simulink model "VSI_SPWM_FOC"  (R2020b)
settings: Solver=FixedStepDiscrete  StartTime=0.0  StopTime=0.02  RelTol=1e-3
libraries: powerlib x16, pid_lib x3, simulink x3, powerlib_meascontrol x1
settings Model: Creator=90554  LastModifiedBy=90554

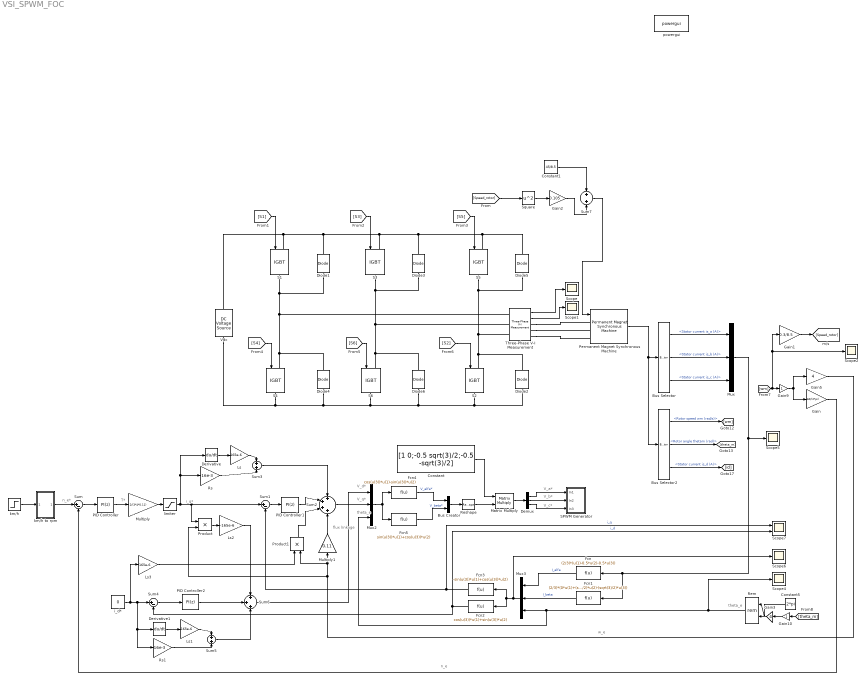
== system VSI_SPWM_FOC ==
  note: V_c*
  note: V_b*
  note: V_a*
  note: theta_e
  note: flux linkage
  note: n_e*
  note: T*
  note: i_q*
  note: V_q*
  note: V_d*
  note: n_e
  note: w_e
  note: theta_e
  Bus Creator : BusCreator  Inputs=2
  Bus Selector : BusSelector  OutputSignals=Stator current is_a (A),Stator current is_b (A),Stator current is_c (A)
  Bus Selector2 : BusSelector  OutputSignals=Rotor speed wm (rad/s),Rotor angle thetam (rad),Stator current is_d (A)
  Constant : Constant  Value=[1 0;-0.5 sqrt(3)/2;-0.5 -sqrt(3)/2]  VectorParams1D=off
  Constant1 : Constant  Value=45/8.5
  Constant5 : Constant  Value=2*pi
  Demux : Demux  Outputs=3
  Derivative : Derivative
  Derivative1 : Derivative
  Diode{1..6} (6 alike) : powerlib/Power Electronics/Diode  Ron=0.001  Lon=0  Vf=0.8  IC=0  UseSnubber=0  Rs=inf  Cs=0  Measurements=off
  Fcn : Fcn  Expr=(2/3)*(u(1)-0.5*u(2)-0.5*u(3))
  Fcn1 : Fcn  Expr=(2/3)*(0*u(1)+(sqrt(3)/2)*u(2)-(sqrt(3)/2)*u(3))
  Fcn2 : Fcn  Expr=cos(u(3))*u(1)+sin(u(3))*u(2)
  Fcn3 : Fcn  Expr=-sin(u(3))*u(1)+cos(u(3))*u(2)
  Fcn4 : Fcn  Expr=cos(u(3))*u(1)-sin(u(3))*u(2)
  Fcn5 : Fcn  Expr=sin(u(3))*u(1)+cos(u(3))*u(2)
  Gain : Gain  Gain=60/(2*pi)
  Gain1 : Gain  Gain=0.3/8.5
  Gain10 : Gain
  Gain2 : Gain  Gain=0.105
  Gain3 : Gain  Gain=4
  Gain5 : Gain  Gain=4
  Gain9 : Gain
  Ls : Gain  Gain=165e-6
  Ls1 : Gain  Gain=165e-6
  Ls2 : Gain  Gain=-165e-6
  Ls3 : Gain  Gain=165e-6
  Matrix Multiply : Product  Multiplication=Matrix(*)
  Multiply : Gain  Gain=2/(3*4*0.11)
  Multiply1 : Gain  Gain=0.11
  Mux : Mux  Inputs=3
  Mux2 : Mux  Inputs=3
  Mux3 : Mux  Inputs=3
  PID Controller : pid_lib/PID Controller  Controller=PI  Form=Parallel  TimeDomain=Discrete-time  UseExternalTs=off  SampleTime=-1  IntegratorMethod=Forward Euler  FilterMethod=Forward Euler  ControllerParametersSource=internal  P=5  I=1  D=0  UseFilter=on  N=100  TunerSelectOption=Transfer Function Based (PID Tuner App)  InitialConditionSource=internal  InitialConditionForIntegrator=0  InitialConditionForFilter=0  DifferentiatorICPrevScaledInput=0  ExternalReset=none  TrackingMode=off  Kt=1  LimitOutput=off  SatLimitsSource=internal  UpperSaturationLimit=inf  LowerSaturationLimit=-inf  LinearizeAsGain=on  AntiWindupMode=none  Kb=1  POutMin=[]  POutMax=[]  IOutMin=[]  IOutMax=[]  DOutMin=[]  DOutMax=[]  NOutMin=[]  NOutMax=[]  SumOutMin=[]  SumOutMax=[]  SaturationOutMin=[]  SaturationOutMax=[]  PParamMin=[]  PParamMax=[]  IParamMin=[]  IParamMax=[]  DParamMin=[]  DParamMax=[]  NParamMin=[]  NParamMax=[]  KbParamMin=[]  KbParamMax=[]  KtParamMin=[]  KtParamMax=[]  KbOutMin=[]  KbOutMax=[]  KtOutMin=[]  KtOutMax=[]  IntegratorOutMin=[]  IntegratorOutMax=[]  FilterOutMin=[]  FilterOutMax=[]  SumI1OutMin=[]  SumI1OutMax=[]  SumI2OutMin=[]  SumI2OutMax=[]  SumI3OutMin=[]  SumI3OutMax=[]  SumI4OutMin=[]  SumI4OutMax=[]  SumDOutMin=[]  SumDOutMax=[]  DifferentiatorOutMin=[]  DifferentiatorOutMax=[]  FilterDiffOutCoefMin=[]  FilterDiffOutCoefMax=[]  ReciprocalOutMin=[]  ReciprocalOutMax=[]  SumDenOutMin=[]  SumDenOutMax=[]  SumNumOutMin=[]  SumNumOutMax=[]  DivideOutMin=[]  DivideOutMax=[]  UdiffTsProdOutMin=[]  UdiffTsProdOutMax=[]  NTsProdOutMin=[]  NTsProdOutMax=[]  UintegralTsProdOutMin=[]  UintegralTsProdOutMax=[]  UngainTsProdOutMin=[]  UngainTsProdOutMax=[]  IntegratorContinuousStateAttributes=''  IntegratorStateMustResolveToSignalObject=off  IntegratorRTWStateStorageClass=Auto  FilterContinuousStateAttributes=''  FilterStateMustResolveToSignalObject=off  FilterRTWStateStorageClass=Auto  ParallelPVariant=InternalParameters  IdealPVariant=Disabled  IVariant=InternalParameters  DVariant=Disabled  IntegratorVariant=Discrete  SatVariant=Disabled  AWVariant=Passthrough  PCopyVariant=Disabled  TRVariant=Disabled  FdbkBlocksVariant=Forward  IdealPFdbkVariant=Disabled  SatFdbkVariant=Disabled  DerivativeFilterVariant=Disabled  NVariant=Disabled  NCopyVariant=Disabled_SignalSpec  FilterICVariant=Disabled  IntegratorICVariant=InternalICs  ExternalResetVariant=Disabled  TRSumVariant=Passthrough  SumFdbkVariant=Disabled  SumVariant=Sum_PI  TsampFilterVariant=InternalTs  TsampNgainVariant=Passthrough  TsampIntegralVariant=Passthrough  ExternalSaturationOutDataTypeStr=Inherit: Same as second input
  PID Controller1 : pid_lib/PID Controller  Controller=PI  Form=Parallel  TimeDomain=Discrete-time  UseExternalTs=off  SampleTime=-1  IntegratorMethod=Forward Euler  FilterMethod=Forward Euler  ControllerParametersSource=internal  P=5  I=1  D=0  UseFilter=on  N=100  TunerSelectOption=Transfer Function Based (PID Tuner App)  InitialConditionSource=internal  InitialConditionForIntegrator=0  InitialConditionForFilter=0  DifferentiatorICPrevScaledInput=0  ExternalReset=none  TrackingMode=off  Kt=1  LimitOutput=off  SatLimitsSource=internal  UpperSaturationLimit=inf  LowerSaturationLimit=-inf  LinearizeAsGain=on  AntiWindupMode=none  Kb=1  POutMin=[]  POutMax=[]  IOutMin=[]  IOutMax=[]  DOutMin=[]  DOutMax=[]  NOutMin=[]  NOutMax=[]  SumOutMin=[]  SumOutMax=[]  SaturationOutMin=[]  SaturationOutMax=[]  PParamMin=[]  PParamMax=[]  IParamMin=[]  IParamMax=[]  DParamMin=[]  DParamMax=[]  NParamMin=[]  NParamMax=[]  KbParamMin=[]  KbParamMax=[]  KtParamMin=[]  KtParamMax=[]  KbOutMin=[]  KbOutMax=[]  KtOutMin=[]  KtOutMax=[]  IntegratorOutMin=[]  IntegratorOutMax=[]  FilterOutMin=[]  FilterOutMax=[]  SumI1OutMin=[]  SumI1OutMax=[]  SumI2OutMin=[]  SumI2OutMax=[]  SumI3OutMin=[]  SumI3OutMax=[]  SumI4OutMin=[]  SumI4OutMax=[]  SumDOutMin=[]  SumDOutMax=[]  DifferentiatorOutMin=[]  DifferentiatorOutMax=[]  FilterDiffOutCoefMin=[]  FilterDiffOutCoefMax=[]  ReciprocalOutMin=[]  ReciprocalOutMax=[]  SumDenOutMin=[]  SumDenOutMax=[]  SumNumOutMin=[]  SumNumOutMax=[]  DivideOutMin=[]  DivideOutMax=[]  UdiffTsProdOutMin=[]  UdiffTsProdOutMax=[]  NTsProdOutMin=[]  NTsProdOutMax=[]  UintegralTsProdOutMin=[]  UintegralTsProdOutMax=[]  UngainTsProdOutMin=[]  UngainTsProdOutMax=[]  IntegratorContinuousStateAttributes=''  IntegratorStateMustResolveToSignalObject=off  IntegratorRTWStateStorageClass=Auto  FilterContinuousStateAttributes=''  FilterStateMustResolveToSignalObject=off  FilterRTWStateStorageClass=Auto  ParallelPVariant=InternalParameters  IdealPVariant=Disabled  IVariant=InternalParameters  DVariant=Disabled  IntegratorVariant=Discrete  SatVariant=Disabled  AWVariant=Passthrough  PCopyVariant=Disabled  TRVariant=Disabled  FdbkBlocksVariant=Forward  IdealPFdbkVariant=Disabled  SatFdbkVariant=Disabled  DerivativeFilterVariant=Disabled  NVariant=Disabled  NCopyVariant=Disabled_SignalSpec  FilterICVariant=Disabled  IntegratorICVariant=InternalICs  ExternalResetVariant=Disabled  TRSumVariant=Passthrough  SumFdbkVariant=Disabled  SumVariant=Sum_PI  TsampFilterVariant=InternalTs  TsampNgainVariant=Passthrough  TsampIntegralVariant=Passthrough  ExternalSaturationOutDataTypeStr=Inherit: Same as second input
  PID Controller2 : pid_lib/PID Controller  Controller=PI  Form=Parallel  TimeDomain=Discrete-time  UseExternalTs=off  SampleTime=-1  IntegratorMethod=Forward Euler  FilterMethod=Forward Euler  ControllerParametersSource=internal  P=5  I=1  D=0  UseFilter=on  N=100  TunerSelectOption=Transfer Function Based (PID Tuner App)  InitialConditionSource=internal  InitialConditionForIntegrator=0  InitialConditionForFilter=0  DifferentiatorICPrevScaledInput=0  ExternalReset=none  TrackingMode=off  Kt=1  LimitOutput=off  SatLimitsSource=internal  UpperSaturationLimit=inf  LowerSaturationLimit=-inf  LinearizeAsGain=on  AntiWindupMode=none  Kb=1  POutMin=[]  POutMax=[]  IOutMin=[]  IOutMax=[]  DOutMin=[]  DOutMax=[]  NOutMin=[]  NOutMax=[]  SumOutMin=[]  SumOutMax=[]  SaturationOutMin=[]  SaturationOutMax=[]  PParamMin=[]  PParamMax=[]  IParamMin=[]  IParamMax=[]  DParamMin=[]  DParamMax=[]  NParamMin=[]  NParamMax=[]  KbParamMin=[]  KbParamMax=[]  KtParamMin=[]  KtParamMax=[]  KbOutMin=[]  KbOutMax=[]  KtOutMin=[]  KtOutMax=[]  IntegratorOutMin=[]  IntegratorOutMax=[]  FilterOutMin=[]  FilterOutMax=[]  SumI1OutMin=[]  SumI1OutMax=[]  SumI2OutMin=[]  SumI2OutMax=[]  SumI3OutMin=[]  SumI3OutMax=[]  SumI4OutMin=[]  SumI4OutMax=[]  SumDOutMin=[]  SumDOutMax=[]  DifferentiatorOutMin=[]  DifferentiatorOutMax=[]  FilterDiffOutCoefMin=[]  FilterDiffOutCoefMax=[]  ReciprocalOutMin=[]  ReciprocalOutMax=[]  SumDenOutMin=[]  SumDenOutMax=[]  SumNumOutMin=[]  SumNumOutMax=[]  DivideOutMin=[]  DivideOutMax=[]  UdiffTsProdOutMin=[]  UdiffTsProdOutMax=[]  NTsProdOutMin=[]  NTsProdOutMax=[]  UintegralTsProdOutMin=[]  UintegralTsProdOutMax=[]  UngainTsProdOutMin=[]  UngainTsProdOutMax=[]  IntegratorContinuousStateAttributes=''  IntegratorStateMustResolveToSignalObject=off  IntegratorRTWStateStorageClass=Auto  FilterContinuousStateAttributes=''  FilterStateMustResolveToSignalObject=off  FilterRTWStateStorageClass=Auto  ParallelPVariant=InternalParameters  IdealPVariant=Disabled  IVariant=InternalParameters  DVariant=Disabled  IntegratorVariant=Discrete  SatVariant=Disabled  AWVariant=Passthrough  PCopyVariant=Disabled  TRVariant=Disabled  FdbkBlocksVariant=Forward  IdealPFdbkVariant=Disabled  SatFdbkVariant=Disabled  DerivativeFilterVariant=Disabled  NVariant=Disabled  NCopyVariant=Disabled_SignalSpec  FilterICVariant=Disabled  IntegratorICVariant=InternalICs  ExternalResetVariant=Disabled  TRSumVariant=Passthrough  SumFdbkVariant=Disabled  SumVariant=Sum_PI  TsampFilterVariant=InternalTs  TsampNgainVariant=Passthrough  TsampIntegralVariant=Passthrough  ExternalSaturationOutDataTypeStr=Inherit: Same as second input
  Permanent Magnet Synchronous Machine : powerlib/Machines/Permanent Magnet Synchronous Machine  NbPhases=3  FluxDistribution=Sinusoidal  RotorType=Round  MechanicalLoad=Torque Tm  PresetModel=No  ShowDetailedParameters=on  MeasurementBus=off  Resistance=16e-3  Inductance=8.5e-3  dqInductances=[8.5e-3,8.5e-3]  La=165e-6  MachineConstant=Flux linkage established by magnets (V.s)  Flux=0.11  VoltageCst=79.8072  TorqueCst=0.66  Flat=120  Mechanical=[2.4232 0 4 0]  PolePairs=4  InitialConditions=[0,0, 0,0]  InitialConditions5ph=[0 0 0 0 0 0]  RefAngle=Aligned with phase A axis (original Park)  IterativeDiscreteModel=Trapezoidal non iterative  TsBlock=-1  TsPowergui=0
  Product : Product
  Product1 : Product
  Rem : Math  Operator=rem  SignedPower=on  SaturateOnIntegerOverflow=on
  Reshape : Reshape  OutputDimensionality=Column vector (2-D)
  Rs : Gain  Gain=16e-3
  Rs1 : Gain  Gain=16e-3
  S{1..6} (6 alike) : powerlib/Power Electronics/IGBT  Ron=0.001  Lon=0  Vf=1  Tf=1e-6  Tt=2e-6  IC=0  Rs=1e5  Cs=inf  Measurements=off
  SPWM Generator : Subsystem
  Scope{,1..2,4..6} (6 alike) : Scope
  Scope7 : Scope  NumInputPorts=2
  Square : Math  Operator=square  SaturateOnIntegerOverflow=on
  Sum : Sum  Inputs=|+-
  Sum1 : Sum  Inputs=|+-
  Sum2 : Sum  Inputs=+|+|+|+
  Sum3 : Sum  Inputs=+|+
  Sum4 : Sum  Inputs=|+-
  Sum5 : Sum  Inputs=+|+
  Sum6 : Sum  Inputs=+|+|+
  Sum7 : Sum  Inputs=+|+
  Three-Phase V-I Measurement : powerlib/Measurements/Three-Phase V-I Measurement  VoltageMeasurement=phase-to-phase  SetLabelV=off  LabelV=Vabc  Vpu=off  VpuLL=off  CurrentMeasurement=yes  SetLabelI=off  LabelI=Iabc  Ipu=off  Pbase=100e6  Vbase=500e3  OutputType=Complex  PhasorSimulation=off  PSBequivalent=0
  Vdc : powerlib/Electrical Sources/DC Voltage Source  Amplitude=420  Measurements=Voltage
  i_d* : Constant  Value=0
  km/h : Step  Time=5  Before=35  After=40  SampleTime=0
  km/h to rpm : Subsystem
  limiter : Saturate  UpperLimit=500  LowerLimit=0
  powergui : powerlib/powergui  Priority=1  SimulationMode=Discrete  SampleTime=1e-6  frequency=60  Iterations=50  frequencyindice=0  Pbase=100e6  ErrMax=1e-4  UnitsV=kV  UnitsW=MW  buscounter=0  FunctionMessages=off  echomessages=off  EnableUseOfTLC=off  CurrentSourceSwitches=off  DisableSnubberDevices=off  DisableRonSwitches=off  DisableVfSwitches=off  DisplayEquations=off  AutomaticDiscreteSolvers=off  SolverType=Tustin/Backward Euler (TBE)  Interpol=off  ExternalGateDelay=off  methode=off  Ts=100  x0status=blocks  SPID=on  SwTol=0  HookPort=off  NonlinearTolerance=1e-4  nMaxIteration=100  ContinueOnMaxIteration=off  RestoreLinks=warning  ResistiveCurrentMeasurement=off  Frange=[0:2:500]  Ylog=off  Xlog=on  ShowGrid=off  save=off  variable=ZData  structure=0  ZoomFFT=off  StartTime=0.0  cycles=1  DisplayStyle=1  fundamental=60  FreqAxis=off  MaxFrequency=1000  frequencyindicesteady=1  RmsSteady=1  display=off
  wires:
  [S1] -> S1/1
  [S3] -> S3/1
  [S5] -> S5/1
  [S4] -> S4/1
  [S6] -> S6/1
  [S2] -> S2/1
  km/h/1 -> km/h to rpm/1(In1)
  km/h to rpm/1(Out1) -> Sum/1
  Sum/1 -> PID Controller/1
  PID Controller/1 -> Multiply/1
  Multiply/1 -> limiter/1
  Derivative/1 -> Ls/1
  limiter/1 -> Sum1/1, Product/1, Rs/1, Derivative/1
  Sum1/1 -> PID Controller1/1
  Ls/1 -> Sum3/1
  Rs/1 -> Sum3/2
  PID Controller1/1 -> Sum2/2
  Sum3/1 -> Sum2/1
  Bus Creator/1 -> Reshape/1
  Reshape/1 -> Matrix Multiply/2
  Bus Selector/2 -> Mux/2  "<Stator current is_b (A)>"
  Permanent Magnet Synchronous Machine/1 -> Bus Selector2/1, Bus Selector/1
  Bus Selector2/2 -> [theta_m]  "<Rotor angle thetam (rad)>"
  Gain10/1 -> Gain3/1
  [theta_m] -> Gain10/1
  Gain9/1 -> Gain/1, Gain5/1
  [wm] -> Scope2/1, Gain1/1, Gain9/1
  Gain/1 -> Sum/2
  Constant5/1 -> Rem/2
  Gain3/1 -> Rem/1
  Fcn5/1 -> Bus Creator/2  "V_beta*"
  Sum2/1 -> Mux2/2
  Fcn4/1 -> Bus Creator/1  "V_alfa*"
  Rem/1 -> Scope4/1, Mux2/3, Mux3/3
  Mux2/1 -> Fcn4/1, Fcn5/1
  Constant/1 -> Matrix Multiply/1
  Matrix Multiply/1 -> Demux/1
  Demux/1 -> SPWM Generator/1(In1)
  Demux/2 -> SPWM Generator/2(In2)
  Demux/3 -> SPWM Generator/3(In3)
  Bus Selector2/1 -> [wm]  "<Rotor speed wm (rad/s)>"
  Bus Selector2/3 -> [id]  "<Stator current is_d (A)>"
  Three-Phase V-I Measurement/1 -> Scope/1
  Three-Phase V-I Measurement/2 -> Scope1/1
  Bus Selector/1 -> Mux/1  "<Stator current is_a (A)>"
  Bus Selector/3 -> Mux/3  "<Stator current is_c (A)>"
  Fcn/1 -> Mux3/1  "I_alfa"
  Fcn1/1 -> Mux3/2  "I_beta"
  Fcn3/1 -> Sum1/2, Scope7/1  "i_q"
  Fcn2/1 -> Sum4/2, Scope7/2  "i_d"
  Mux3/1 -> Scope6/1, Fcn3/1, Fcn2/1
  Mux/1 -> Scope5/1, Fcn1/1, Fcn/1
  i_d*/1 -> Ls3/1, Rs1/1, Derivative1/1, Sum4/1
  Sum4/1 -> PID Controller2/1
  Rs1/1 -> Sum5/2
  Ls1/1 -> Sum5/1
  Derivative1/1 -> Ls1/1
  Sum5/1 -> Sum6/3
  PID Controller2/1 -> Sum6/2
  Gain5/1 -> Product/2, Product1/2, Multiply1/1
  Product/1 -> Ls2/1
  Ls2/1 -> Sum6/1
  Sum6/1 -> Mux2/1
  Multiply1/1 -> Sum2/4
  Ls3/1 -> Product1/1
  Product1/1 -> Sum2/3
  [Speed_rotor] -> Square/1
  Square/1 -> Gain2/1
  Gain2/1 -> Sum7/2
  Constant1/1 -> Sum7/1
  Sum7/1 -> Permanent Magnet Synchronous Machine/1
  Gain1/1 -> [Speed_rotor]
  connections:
  S4/LConn1 -- Diode4/RConn1 -- Three-Phase V-I Measurement/LConn1 -- Diode1/LConn1 -- S1/RConn1
  S3/RConn1 -- Diode3/LConn1 -- Three-Phase V-I Measurement/LConn2 -- Diode6/RConn1 -- S6/LConn1
  S5/RConn1 -- Diode5/LConn1 -- Three-Phase V-I Measurement/LConn3 -- Diode2/RConn1 -- S2/LConn1
  Vdc/RConn1 -- S1/LConn1 -- Diode1/RConn1 -- S3/LConn1 -- Diode3/RConn1 -- S5/LConn1 -- Diode5/RConn1
  Vdc/LConn1 -- S4/RConn1 -- Diode4/LConn1 -- S6/RConn1 -- Diode6/LConn1 -- S2/RConn1 -- Diode2/LConn1
  Three-Phase V-I Measurement/RConn1 -- Permanent Magnet Synchronous Machine/LConn1
  Three-Phase V-I Measurement/RConn2 -- Permanent Magnet Synchronous Machine/LConn2
  Three-Phase V-I Measurement/RConn3 -- Permanent Magnet Synchronous Machine/LConn3

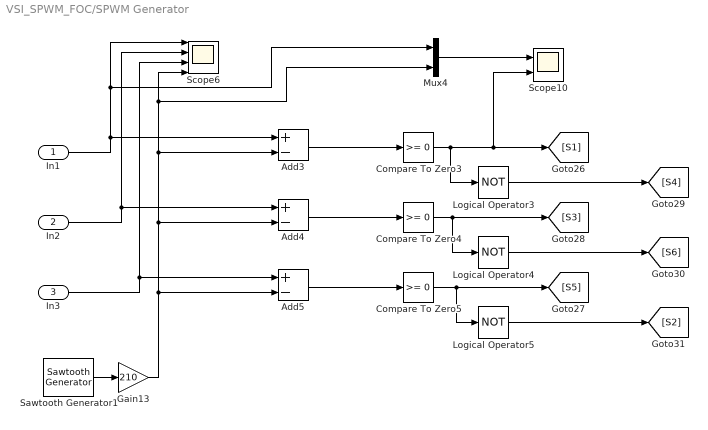
== system VSI_SPWM_FOC/SPWM Generator ==
  In1 : Inport
  In2 : Inport  Port=2
  In3 : Inport  Port=3
  Add3 : Sum  Inputs=+-
  Add4 : Sum  Inputs=+-
  Add5 : Sum  Inputs=+-
  Compare To Zero3 : simulink/Logic and Bit Operations/Compare To Zero  relop=>=  OutDataTypeStr=boolean
  Compare To Zero4 : simulink/Logic and Bit Operations/Compare To Zero  relop=>=  OutDataTypeStr=boolean
  Compare To Zero5 : simulink/Logic and Bit Operations/Compare To Zero  relop=>=  OutDataTypeStr=boolean
  Gain13 : Gain  Gain=210
  Logical Operator3 : Logic  Operator=NOT  AllPortsSameDT=off  OutDataTypeStr=boolean
  Logical Operator4 : Logic  Operator=NOT  AllPortsSameDT=off  OutDataTypeStr=boolean
  Logical Operator5 : Logic  Operator=NOT  AllPortsSameDT=off  OutDataTypeStr=boolean
  Mux4 : Mux  Inputs=2
  Sawtooth Generator1 : powerlib_meascontrol/Pulse & Signal Generators/Sawtooth Generator  Freq=10e3  Phase=180  Ts=0
  Scope10 : Scope  NumInputPorts=2
  Scope6 : Scope  NumInputPorts=4
  wires:
  Compare To Zero5/1 -> Logical Operator5/1, [S5]
  Logical Operator3/1 -> [S4]
  In1/1 -> Add3/1, Scope6/1, Mux4/1
  Compare To Zero4/1 -> Logical Operator4/1, [S3]
  Compare To Zero3/1 -> Logical Operator3/1, [S1], Scope10/2
  Add3/1 -> Compare To Zero3/1
  Gain13/1 -> Add5/2, Add4/2, Add3/2, Mux4/2, Scope6/4
  In2/1 -> Scope6/2, Add4/1
  Mux4/1 -> Scope10/1
  Logical Operator4/1 -> [S6]
  Sawtooth Generator1/1 -> Gain13/1
  Add4/1 -> Compare To Zero4/1
  In3/1 -> Add5/1, Scope6/3
  Logical Operator5/1 -> [S2]
  Add5/1 -> Compare To Zero5/1

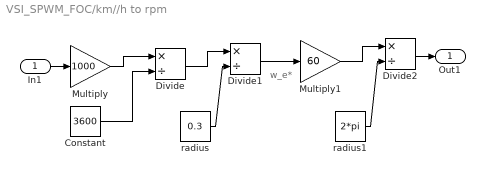
== system VSI_SPWM_FOC/km//h to rpm ==
  note: w_e*
  In1 : Inport
  Constant : Constant  Value=3600
  Divide : Product  Inputs=*/
  Divide1 : Product  Inputs=*/
  Divide2 : Product  Inputs=*/
  Multiply : Gain  Gain=1000
  Multiply1 : Gain  Gain=60
  radius : Constant  Value=0.3
  radius1 : Constant  Value=2*pi
  Out1 : Outport
  wires:
  Multiply/1 -> Divide/1
  Constant/1 -> Divide/2
  radius/1 -> Divide1/2
  Divide1/1 -> Multiply1/1
  radius1/1 -> Divide2/2
  Multiply1/1 -> Divide2/1
  Divide2/1 -> Out1/1
  In1/1 -> Multiply/1
  Divide/1 -> Divide1/1
